simulink model "TestRocket_2026"  (R2025a)
settings: Solver=VariableStepAuto  StartTime=0.0  StopTime=10.0  RelTol=1e-3
libraries: aerolibasang x3, simulink_extras x1, aerolibatmos2 x1
settings Model: Creator=Ranvir  LastModifiedBy=Ranvir

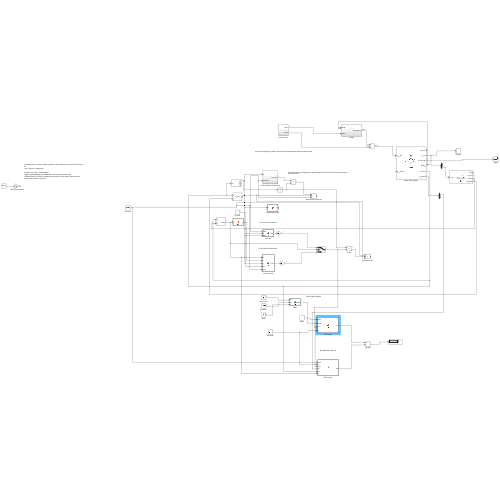
[thumbnail: Simulink's stored preview of the top-level diagram]
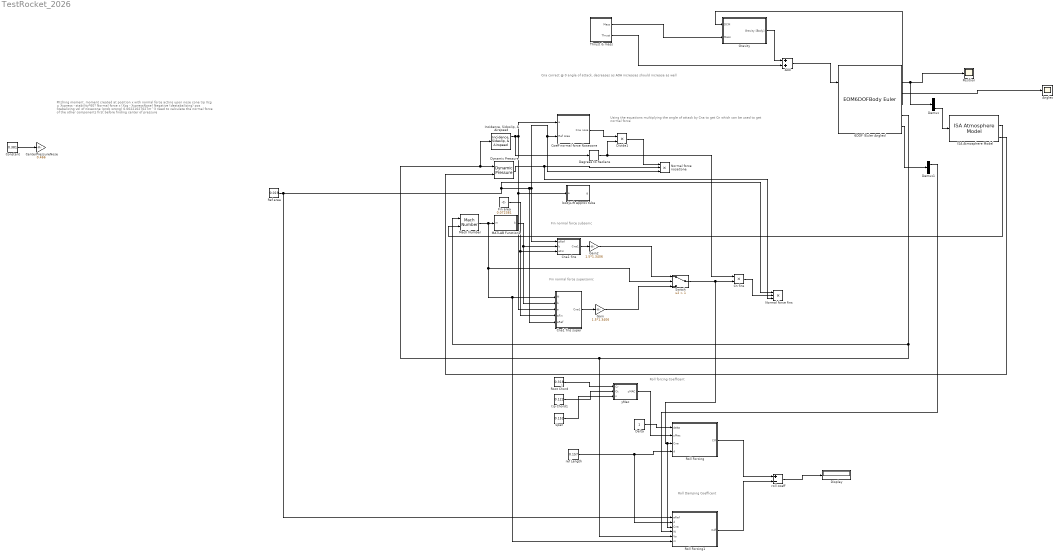
== system TestRocket_2026 ==
  note: 1
  note: Roll forcing Coefficent
  note: Fin normal force supersonic
  note: Pitching moment, moment created at position x with normal force acting upon nose cone tip
      | Xcg = Xcpress - stability*60?
      |
      | Normal force x (Xcg - XcpressNose)
      | Negative (destabalizing) pos Stabalizing vol of nosecone (prob wrong) 0.00221027027m^3 need to calculate the normal force of the other components first before finding center of pressure
  note: Using the equations multiplying the angle of attack by Cna to get Cn which can be used to get normal force
  note: Cna correct @ 0 angle of attack, decreases as AOA increases should increase as well
  note: Fin normal force subsonic
  note: Roll Damping Coefficent
  6DOF (Euler Angles) : EOM6DOFBodyEuler  mass_0=26.452  inertia=[6.531914 0 0; 0 6.531914 0; 0 0 0.635615]
  Add : Sum
  Angles : Scope
      settings: ActiveDisplayYMinimum=-1  ActiveDisplayYMaximum=1
  CenterPressureNose : Gain  Gain=0.466
  Cn fins : Product  Inputs=**
  Cna1 fins : MATLAB Function  TreatAsAtomicUnit=on
  Cna1 fins super : MATLAB Function  TreatAsAtomicUnit=on
  Coeff normal force Nosecone : Subsystem
  Constant : Constant  Value=0.381
  Degrees to Radians : simulink_extras/Transformations/Degrees to Radians
  Delta : Constant
  Demux : Demux  Outputs=3
  Demux1 : Demux  Outputs=3
  Display : Display
  Divide1 : Product  Inputs=**
  Dynamic Pressure : aerolibasang/Dynamic Pressure
  Fin area : Constant  Value=0.072381
  Gain : Gain  Gain=1.5*1.3406
  Gain2 : Gain  Gain=1.5*1.3406
  Gravity : Subsystem
  ISA Atmosphere Model : aerolibatmos2/ISA Atmosphere Model  useExtended=off  action=None  custom=off  viscosityOut=off  g=9.80665  gamma=1.4  R=287.0531  L=0.0065  h_trop=11000  h_strat=20000  rho0=1.225  P0=101325  T0=288.15  h0=0  S=110.4  Tref=273.15  muref=1.716e-5
  "Incidence, Sideslip, & Airspeed" : aerolibasang/Incidence, Sideslip, & Airspeed
  MATLAB Function1 : MATLAB Function  TreatAsAtomicUnit=on
  Mach Number : aerolibasang/Mach Number
  Normal force fins : Product  Inputs=***
  Normal force noseCone : Product  Inputs=***
  Position : Scope
      settings: ActiveDisplayYMinimum=-1  ActiveDisplayYMaximum=1
  Ref area : Constant  Value=0.019
  Roll Forcing : MATLAB Function  TreatAsAtomicUnit=on
  Roll Forcing1 : MATLAB Function  TreatAsAtomicUnit=on
  Root Chord : Constant  Value=0.318
  Span : Constant  Value=0.152
  Switch : Switch  Criteria=u2 > Threshold  Threshold=1  SaturateOnIntegerOverflow=off  InputSameDT=off
  Thrust & mass : Subsystem
  bodyLift Approx tube : MATLAB Function  TreatAsAtomicUnit=on
  ref Length : Constant  Value=0.157
  roll coeff : Sum  Inputs=+-
  tip Chord1 : Constant  Value=0.122
  yMac : MATLAB Function  TreatAsAtomicUnit=on
  wires:
  6DOF (Euler Angles)/4 -> Gravity/1(DCM)
  Thrust & mass/1(Mass) -> Gravity/2(Mass)
  Gravity/1(Gravity [Body]) -> Add/1
  Thrust & mass/2(Thrust) -> Add/2
  Add/1 -> 6DOF (Euler Angles)/1
  6DOF (Euler Angles)/2 -> Demux/1, Position/1
  6DOF (Euler Angles)/3 -> Angles/1
  "Incidence, Sideslip, & Airspeed"/1 -> Cna1 fins super/3(a), bodyLift Approx tube/1(a), Coeff normal force Nosecone/1(a), Degrees to Radians/1
  Ref area/1 -> Roll Forcing1/1(aRef), Normal force fins/1, Cna1 fins super/5(aRef), Normal force noseCone/3, Coeff normal force Nosecone/2(Ref Area), Cna1 fins/1(aRef)
  Demux/3 -> ISA Atmosphere Model/1
  6DOF (Euler Angles)/5 -> Mach Number/1, Roll Forcing1/5(Vo), "Incidence, Sideslip, & Airspeed"/1, Dynamic Pressure/1
  ISA Atmosphere Model/4 -> Dynamic Pressure/2
  Dynamic Pressure/1 -> Normal force fins/3, Normal force noseCone/2
  Coeff normal force Nosecone/1(Cna nose) -> Divide1/1
  Divide1/1 -> Normal force noseCone/1
  Degrees to Radians/1 -> Cn fins/1, Divide1/2
  Constant/1 -> CenterPressureNose/1
  ISA Atmosphere Model/2 -> Mach Number/2
  Mach Number/1 -> Switch/2, Roll Forcing1/6(m), Cna1 fins super/1(M), MATLAB Function1/1(m)
  MATLAB Function1/1(b) -> Cna1 fins super/2(b), Cna1 fins/2(b)
  Fin area/1 -> Cna1 fins super/4(aFin), Cna1 fins/3(aFin)
  Cna1 fins super/1(Cna1) -> Gain/1
  Cna1 fins/1(Cna1) -> Gain2/1
  Gain/1 -> Switch/3
  Gain2/1 -> Switch/1
  Switch/1 -> Roll Forcing1/3(Cna), Roll Forcing/3(Cna), Cn fins/2
  Cn fins/1 -> Normal force fins/2
  ref Length/1 -> Roll Forcing1/2(d), Roll Forcing/4(d)
  Delta/1 -> Roll Forcing/1(delta)
  yMac/1(yMAC) -> Roll Forcing/2(yMac)
  Root Chord/1 -> yMac/1(Cr)
  tip Chord1/1 -> yMac/2(Ct)
  Span/1 -> yMac/3(s)
  6DOF (Euler Angles)/6 -> Demux1/1
  Demux1/1 -> Roll Forcing1/4(W)
  Roll Forcing/1(Clf) -> roll coeff/1
  Roll Forcing1/1(Cdf) -> roll coeff/2
  roll coeff/1 -> Display/1

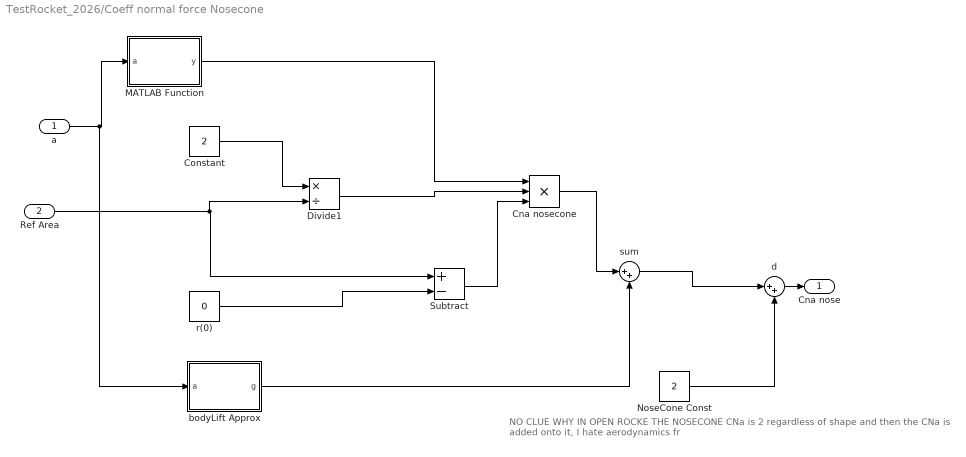
== system TestRocket_2026/Coeff normal force Nosecone ==
  note: NO CLUE WHY IN OPEN ROCKE THE NOSECONE CNa is 2 regardless of shape and then the CNa is added onto it, I hate aerodynamics fr
  a : Inport
  Ref Area : Inport  Port=2
  Cna nosecone : Product  Inputs=***
  Constant : Constant  Value=2
  Divide1 : Product  Inputs=*/
  MATLAB Function : MATLAB Function  TreatAsAtomicUnit=on
  NoseCone Const : Constant  Value=2
  Subtract : Sum  Inputs=+-
  bodyLift Approx : MATLAB Function  TreatAsAtomicUnit=on
  d : Sum  Inputs=|++
  r(0) : Constant  Value=0
  sum : Sum  Inputs=|++
  Cna nose : Outport
  wires:
  Ref Area/1 -> Divide1/2, Subtract/1
  Cna nosecone/1 -> sum/1
  sum/1 -> d/1
  Subtract/1 -> Cna nosecone/3
  bodyLift Approx/1(g) -> sum/2
  Constant/1 -> Divide1/1
  MATLAB Function/1(y) -> Cna nosecone/1
  a/1 -> bodyLift Approx/1(a), MATLAB Function/1(a)
  Divide1/1 -> Cna nosecone/2
  r(0)/1 -> Subtract/2
  NoseCone Const/1 -> d/2
  d/1 -> Cna nose/1

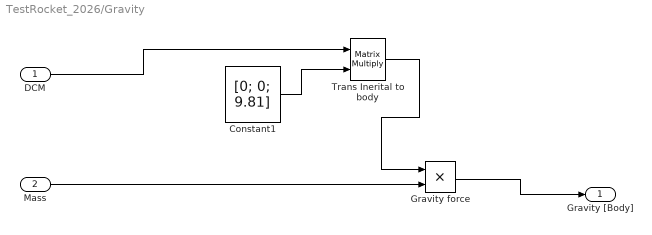
== system TestRocket_2026/Gravity ==
  DCM : Inport
  Mass : Inport  Port=2
  Constant1 : Constant  Value=[0; 0; 9.81]  VectorParams1D=off
  Gravity force : Product  Inputs=**
  Trans Inerital to body : Product  Multiplication=Matrix(*)
  Gravity [Body] : Outport
  wires:
  Constant1/1 -> Trans Inerital to body/2
  Trans Inerital to body/1 -> Gravity force/1
  Mass/1 -> Gravity force/2
  Gravity force/1 -> Gravity [Body]/1
  DCM/1 -> Trans Inerital to body/1

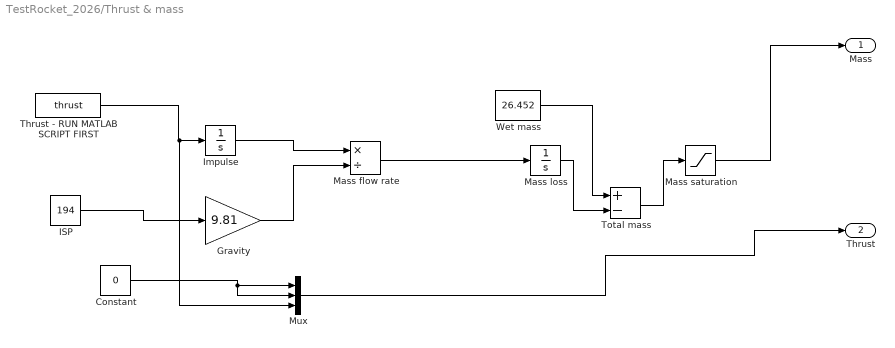
== system TestRocket_2026/Thrust & mass ==
  Constant : Constant  Value=0
  Gravity : Gain  Gain=9.81
  ISP : Constant  Value=194
  Impulse : Integrator
  Mass flow rate : Product  Inputs=*/
  Mass loss : Integrator  UpperSaturationLimit=7  LowerSaturationLimit=0
  Mass saturation : Saturate  UpperLimit=26.452  LowerLimit=19.536
  Mux : Mux  Inputs=3
  Thrust - RUN MATLAB SCRIPT FIRST : FromWorkspace  VariableName=thrust  OutputAfterFinalValue=Setting to zero
  Total mass : Sum  Inputs=+-
  Wet mass : Constant  Value=26.452
  Mass : Outport
  Thrust : Outport  Port=2
  wires:
  Thrust - RUN MATLAB SCRIPT FIRST/1 -> Mux/3, Impulse/1
  Total mass/1 -> Mass saturation/1
  Gravity/1 -> Mass flow rate/2
  Mass flow rate/1 -> Mass loss/1
  Wet mass/1 -> Total mass/1
  ISP/1 -> Gravity/1
  Impulse/1 -> Mass flow rate/1
  Mass loss/1 -> Total mass/2
  Mass saturation/1 -> Mass/1
  Constant/1 -> Mux/2, Mux/1
  Mux/1 -> Thrust/1

== matlab function TestRocket_2026/Coeff normal force Nosecone/bodyLift Approx ==
  data: a input; g output
function g = fcn(a)

g = 1.1*(0.263603/0.019)*sind(a)^2;

== matlab function TestRocket_2026/Coeff normal force Nosecone/MATLAB Function ==
  data: a input; y output
function y = fcn(a)

if a == 0
    y = 1;
else
    y = sind(a)/a;
end

== matlab function TestRocket_2026/bodyLift Approx tube ==
  data: a input; g output
function g = fcn(a)

g = 1.1*(0.263603/0.019)*sind(a)^2;

== matlab function TestRocket_2026/Cna1 fins ==
  data: aRef input; Cna1 output; b input; aFin input
function Cna1 = fcn(aRef, b, aFin)

s = 0.152; %m^2
 %m^2
sA = 30.8; %deg


top = (2*pi) * ((s^2)/aRef);
fd = (b*s^2)/(aFin*cosd(sA)); 
bot = 1+sqrt(1+fd^2);


Cna1 = top/bot;

== matlab function TestRocket_2026/MATLAB Function1 ==
  data: m input; b output
function b = fcn(m)

b = sqrt(abs((m^2) - 1));

== matlab function TestRocket_2026/Cna1 fins super ==
  data: M input; Cna1 output; b input; a input; aFin input; aRef input
function Cna1 = fcn(M, b, a, aFin, aRef)

gam = 1.4;
gam1 = gam+1;

k1 = 2/b;
k2 = (gam1*(M^4) -(4*b^2))/(4*b^4);
k3 = ( (gam1*M^8)  + ((2*gam^2 - 7*gam - 5)*M^6) + 10*(gam1)*M^4 + 8)/(6*b^7);






Cna1 = (aFin/aRef) *(k1 + k2*a + k3*a^2);

== matlab function TestRocket_2026/Roll Forcing ==
  data: delta input; yMac input; Clf output; Cna input; d input
function Clf = fcn(delta, yMac, Cna, d)

rt = 0.0785;
N = 3;

Clf = (N*(yMac + rt)*Cna*delta)/d;

== matlab function TestRocket_2026/yMac ==
  data: Cr input; yMAC output; Ct input; s input
function yMAC = fcn(Cr, Ct, s)




yMAC = (s/3) * ((Cr+2*Ct)/(Cr+Ct));

== matlab function TestRocket_2026/Roll Forcing1 ==
  data: aRef input; d input; Cna input; W input; Cdf output; Vo input; m input
function Cdf = fcn(aRef, d, Cna, W, Vo, m)

rt = 0.0785;
cr = 0.318;
ct = 0.122;
s = 0.152;

v = norm(Vo);

strip = (((cr+ct)/2)*rt^2*s) + (((cr+(2*ct))/3)*rt*s^2) + (((cr+(3*ct))/12)*s^3);



if m >= 1
    Cdf = strip*((3)/(aRef*d));
else
    Cdf = strip*((3*Cna*W)/(aRef*d*v));
end
